simulink model "synchronous_demodulator"  (R2021a)
settings: Solver=VariableStepAuto  StartTime=0.0  StopTime=10.0  RelTol=1e-3
libraries: dsparch4 x1
settings Model: Creator=Fatiha  LastModifiedBy=Fatiha

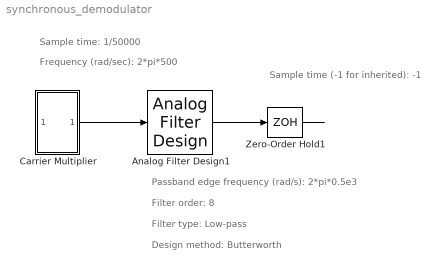
== system synchronous_demodulator ==
  note: Sample time: 1/50000
  note: Frequency (rad/sec): 2*pi*500
  note: Sample time (-1 for inherited): -1
  note: Design method: Butterworth
  note: Filter type: Low-pass
  note: Filter order: 8
  note: Passband edge frequency (rad/s): 2*pi*0.5e3
  Analog Filter Design1 : dsparch4/Analog Filter Design  method=Butterworth  filttype=Lowpass  N=8  Wlo=2*pi*0.5e3  Whi=80  Rp=2  Rs=40
  Carrier Multiplier : Subsystem
  Zero-Order Hold1 : ZeroOrderHold  SampleTime=-1
  wires:
  Analog Filter Design1/1 -> Zero-Order Hold1/1
  Carrier Multiplier/1(Out1) -> Analog Filter Design1/1
  Zero-Order Hold1/1 -> ?
  ? -> Carrier Multiplier/1(In1)

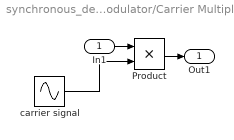
== system synchronous_demodulator/Carrier Multiplier ==
  In1 : Inport
  Product : Product
  carrier signal : Sin  Frequency=2*pi*500  Phase=pi/2  SampleTime=1/50000
  Out1 : Outport
  wires:
  carrier signal/1 -> Product/2
  Product/1 -> Out1/1
  In1/1 -> Product/1
